simulink model "stp1_model"  (R2023b)
settings: Solver=VariableStepAuto  StartTime=0.0  StopTime=t_fin  RelTol=1e-3
InitFcn:
  | simulation_setup
values from neighbouring files (symbols this model uses):
  k = [-20.4 -145.89 -335.994]    [basic_variables.mat]    (also in ex3.m = acker(A, B, sb_vec(i)*ones(1, 3)); ex5.m = acker(A, B, [sb sb sb]); ex6.m = acker(A, B, [sb sb sb]); ex7.m = acker(A, B, [sb sb sb]))
  L = acker(A', C', [s0 s0 s0])    [ex5.m]    (also in ex6.m; ex7.m; simulation_setup.m)
  x_0 = [5 -1 3]    [ex3.m]    (also in ex5.m; ex6.m; ex7.m; extra_ex.m)
  xo_0 = [0 0 0]    [ex5.m]    (also in ex6.m = [10 20 30]; ex7.m = xo_0_vec(i, :); extra_ex.m = [10 20 30]; simulation_setup.m)
settings Model: Creator=piotrpatek  LastModifiedBy=vistek528

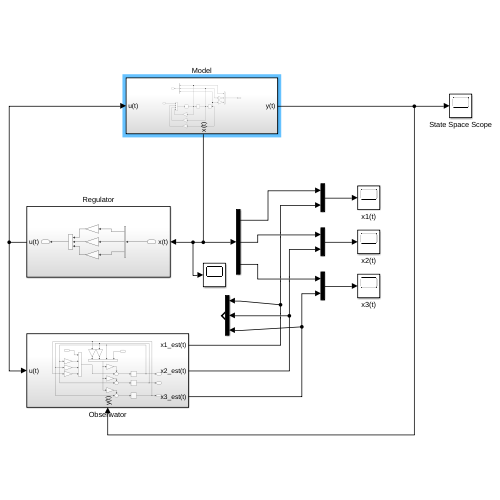
[thumbnail: Simulink's stored preview of the top-level diagram]
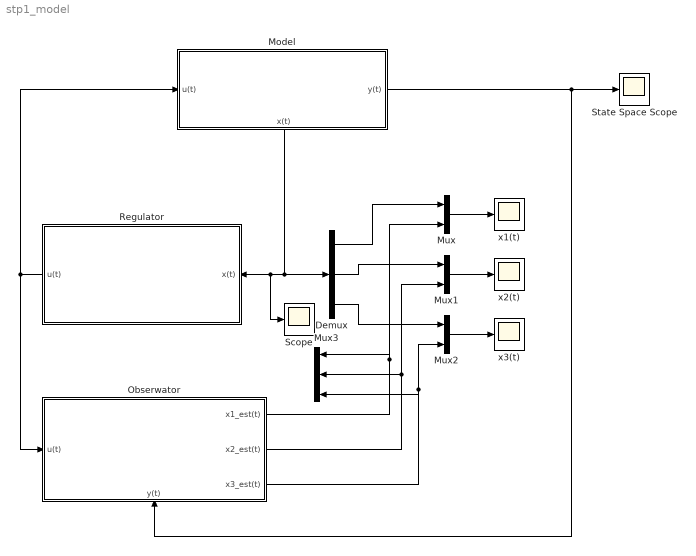
== system stp1_model ==
  Demux : Demux  Outputs=3
  Model : Subsystem
      settings: PortSchema="{\"entries\":[{\"content\":{\"sides\":[{\"content\":{\"connectorIds\":[\"In1\"]},\"type\":\"ConnectorPlacement.EquallySpacedRectSide\",\"uuid\":\"005622f6-1dbe-4fa8-b059-9458e8899b96\"},{\"content\":{\"connectorIds\":[\"Out1\"],\"side\":\"RIGHT\"},\"type\":\"ConnectorPlacement.EquallySpacedRectSide\",\"uuid\":\"7350b0ed-336f-40bc-b296-6ad5a9a87142\"},{\"content\":{\"side\":\"TOP\"},\"type\":\"ConnectorPlacement.EquallySpacedRectSide\",\"uuid\":\"469de851-2f1c-4e76-a936-9009cf2a41ee\"},{\"content\":{\"connectorIds\":[\"Out2\"],\"side\":\"BOTTOM\"},\"type\":\"ConnectorPlacement.EquallySpacedRectSide\",\"uuid\":\"4504609d-b833-4322-8b26-83c28699072e\"}]},\"type\":\"ConnectorPlacement.EquallySpacedConnector\",\"uuid\":\"c3062eda-feb5-4b9f-bf6b-0b995ea2a385\"}],\"packageUris\":[\"http://schema.mathworks.com/mf0/Connector/R2020b\"],\"version\":\"1.0\"}"
  Mux : Mux  Inputs=2
  Mux1 : Mux  Inputs=2
  Mux2 : Mux  Inputs=2
  Mux3 : Mux  Inputs=3
  Obserwator : Subsystem
      settings: PortSchema="{\"entries\":[{\"content\":{\"sides\":[{\"content\":{\"connectorIds\":[\"In1\"]},\"type\":\"ConnectorPlacement.EquallySpacedRectSide\",\"uuid\":\"9b2ff53d-de87-4ad2-b26c-b465d32b1385\"},{\"content\":{\"connectorIds\":[\"Out1\",\"Out2\",\"Out3\"],\"side\":\"RIGHT\"},\"type\":\"ConnectorPlacement.EquallySpacedRectSide\",\"uuid\":\"d6ff340c-c8c1-46fc-9c57-2adcc79a8e31\"},{\"content\":{\"side\":\"TOP\"},\"type\":\"ConnectorPlacement.EquallySpacedRectSide\",\"uuid\":\"f419b5b5-7212-46cf-99f2-e60c41cdc084\"},{\"content\":{\"connectorIds\":[\"In2\"],\"side\":\"BOTTOM\"},\"type\":\"ConnectorPlacement.EquallySpacedRectSide\",\"uuid\":\"27c6ac1b-0d8c-4932-9e64-2403dda0e3e7\"}]},\"type\":\"ConnectorPlacement.EquallySpacedConnector\",\"uuid\":\"cb58852f-7e5f-4311-8779-7dc0488d6073\"}],\"packageUris\":[\"http://schema.mathworks.com/mf0/Connector/R2020b\"],\"version\":\"1.0\"}"
  Regulator : Subsystem
  Scope : Scope
  State Space Scope : Scope
  x1(t) : Scope
  x2(t) : Scope
  x3(t) : Scope
  wires:
  Model/2(x(t)) -> Demux/1, Regulator/1(x(t)), Scope/1
  Regulator/1(u(t)) -> Obserwator/1(u(t)), Model/1(u(t))
  Mux2/1 -> x3(t)/1
  Mux1/1 -> x2(t)/1
  Mux/1 -> x1(t)/1
  Demux/1 -> Mux/1
  Obserwator/1(x1_est(t)) -> Mux3/1, Mux/2
  Demux/2 -> Mux1/1
  Obserwator/2(x2_est(t)) -> Mux3/2, Mux1/2
  Obserwator/3(x3_est(t)) -> Mux3/3, Mux2/2
  Demux/3 -> Mux2/1
  Model/1(y(t)) -> Obserwator/2(y(t)), State Space Scope/1

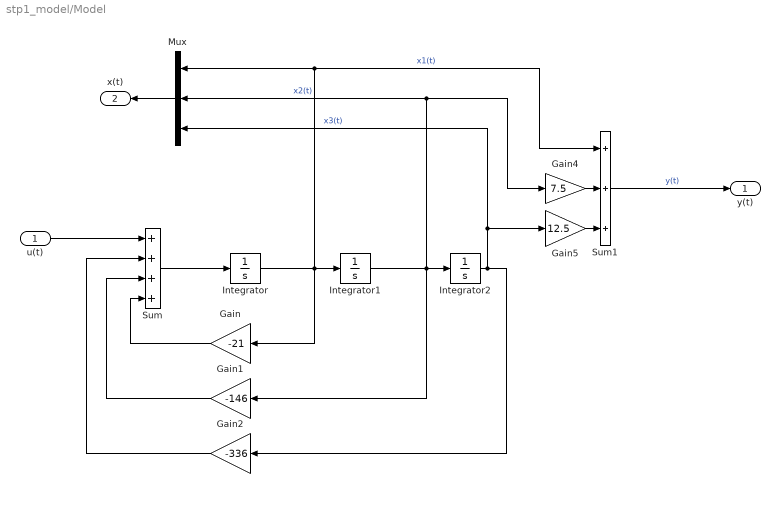
== system stp1_model/Model ==
  u(t) : Inport
  Gain : Gain  Gain=-21
  Gain1 : Gain  Gain=-146
  Gain2 : Gain  Gain=-336
  Gain4 : Gain  Gain=7.5
  Gain5 : Gain  Gain=12.5
  Integrator : Integrator  InitialCondition=x_0(1)
  Integrator1 : Integrator  InitialCondition=x_0(2)
  Integrator2 : Integrator  InitialCondition=x_0(3)
  Mux : Mux  Inputs=3
  Sum : Sum  Inputs=++++
  Sum1 : Sum  Inputs=+++
  y(t) : Outport
  x(t) : Outport  Port=2
  wires:
  Gain5/1 -> Sum1/3
  Gain1/1 -> Sum/3
  Gain2/1 -> Sum/2
  Sum/1 -> Integrator/1
  u(t)/1 -> Sum/1
  Gain4/1 -> Sum1/2
  Sum1/1 -> y(t)/1  "y(t)"
  Gain/1 -> Sum/4
  Integrator/1 -> Gain/1, Mux/1, Sum1/1, Integrator1/1  "x1(t)"
  Integrator2/1 -> Mux/3, Gain5/1, Gain2/1  "x3(t)"
  Integrator1/1 -> Mux/2, Gain4/1, Gain1/1, Integrator2/1  "x2(t)"
  Mux/1 -> x(t)/1

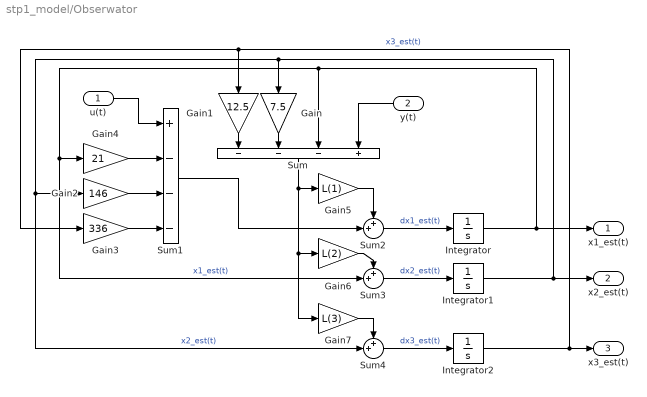
== system stp1_model/Obserwator ==
  u(t) : Inport
  y(t) : Inport  Port=2
  Gain : Gain  Gain=7.5
  Gain1 : Gain  Gain=12.5
  Gain2 : Gain  Gain=146
  Gain3 : Gain  Gain=336
  Gain4 : Gain  Gain=21
  Gain5 : Gain  Gain=L(1)
  Gain6 : Gain  Gain=L(2)
  Gain7 : Gain  Gain=L(3)
  Integrator : Integrator  InitialCondition=xo_0(1)
  Integrator1 : Integrator  InitialCondition=xo_0(2)
  Integrator2 : Integrator  InitialCondition=xo_0(3)
  Sum : Sum  Inputs=---+
  Sum1 : Sum  Inputs=+---
  Sum2 : Sum  Inputs=++|
  Sum3 : Sum  Inputs=++|
  Sum4 : Sum  Inputs=++|
  x1_est(t) : Outport
  x2_est(t) : Outport  Port=2
  x3_est(t) : Outport  Port=3
  wires:
  Gain7/1 -> Sum4/1
  Gain1/1 -> Sum/1
  Gain6/1 -> Sum3/1
  Sum1/1 -> Sum2/2
  Sum2/1 -> Integrator/1  "dx1_est(t)"
  Sum3/1 -> Integrator1/1  "dx2_est(t)"
  Gain2/1 -> Sum1/3
  Integrator/1 -> x1_est(t)/1, Gain4/1, Sum3/2, Sum/3  "x1_est(t)"
  Sum4/1 -> Integrator2/1  "dx3_est(t)"
  Sum/1 -> Gain5/1, Gain6/1, Gain7/1
  Gain/1 -> Sum/2
  Integrator2/1 -> x3_est(t)/1, Gain3/1, Gain1/1  "x3_est(t)"
  Gain3/1 -> Sum1/4
  Integrator1/1 -> x2_est(t)/1, Sum4/2, Gain2/1, Gain/1  "x2_est(t)"
  u(t)/1 -> Sum1/1
  Gain4/1 -> Sum1/2
  Gain5/1 -> Sum2/1
  y(t)/1 -> Sum/4

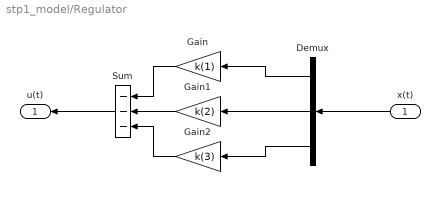
== system stp1_model/Regulator ==
  x(t) : Inport
  Demux : Demux  Outputs=3
  Gain : Gain  Gain=k(1)
  Gain1 : Gain  Gain=k(2)
  Gain2 : Gain  Gain=k(3)
  Sum : Sum  Inputs=---
  u(t) : Outport
  wires:
  Demux/3 -> Gain2/1
  Gain/1 -> Sum/1
  Demux/2 -> Gain1/1
  Gain1/1 -> Sum/2
  x(t)/1 -> Demux/1
  Demux/1 -> Gain/1
  Gain2/1 -> Sum/3
  Sum/1 -> u(t)/1
